simulink model "Filter_data"  (R2025b)
settings: Solver=VariableStepAuto  StartTime=0.0  StopTime=1000  RelTol=1e-3
settings Model: Creator=user  LastModifiedBy=user

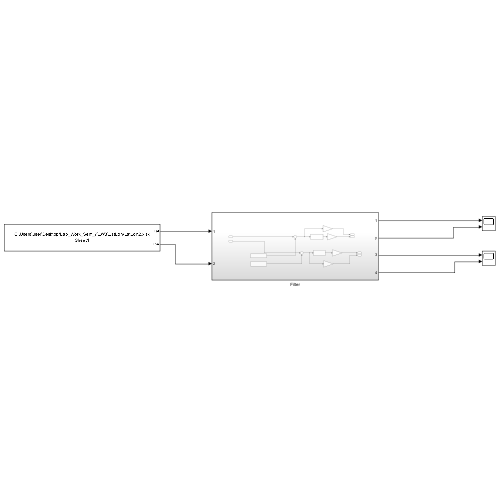
[thumbnail: Simulink's stored preview of the top-level diagram]
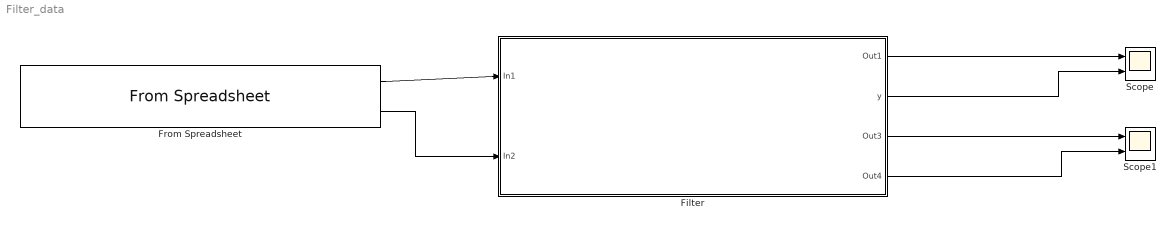
== system Filter_data ==
  Filter : Subsystem
  From Spreadsheet : FromSpreadsheet  FileName=C:\Users\user\Desktop\Lab_Work_Sem_7\LW3\LatLon\LatLon2.xlsx
  Scope : Scope  NumInputPorts=2
      settings: ActiveDisplayYMinimum=-0.22676819893149508  ActiveDisplayYMaximum=2.0409137903834562
  Scope1 : Scope  NumInputPorts=2
      settings: ActiveDisplayYMinimum=-9.25020012785229  ActiveDisplayYMaximum=4.2371666948008748
  wires:
  From Spreadsheet/1 -> Filter/1(In1)
  From Spreadsheet/2 -> Filter/2(In2)
  Filter/1(Out1) -> Scope/1
  Filter/2(y) -> Scope/2
  Filter/3(Out3) -> Scope1/1
  Filter/4(Out4) -> Scope1/2

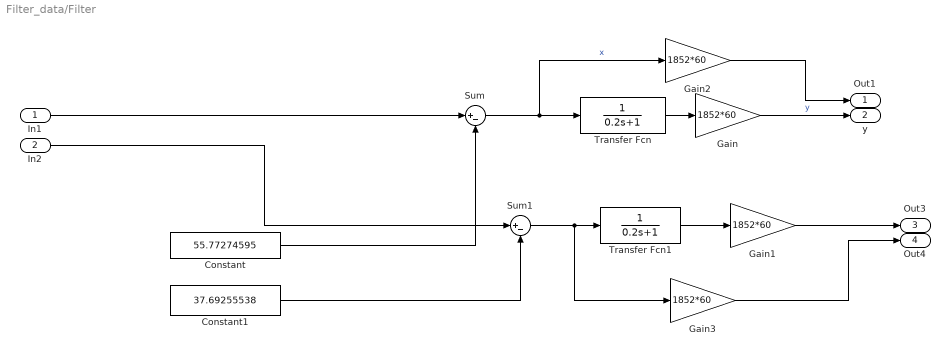
== system Filter_data/Filter ==
  In1 : Inport
  In2 : Inport  Port=2
  Constant : Constant  Value=55.77274595
  Constant1 : Constant  Value=37.69255538
  Gain{,1..3} (4 alike) : Gain  Gain=1852*60
  Sum : Sum  Inputs=|+-
  Sum1 : Sum  Inputs=|+-
  Transfer Fcn : TransferFcn  Denominator=[0.2 1]
  Transfer Fcn1 : TransferFcn  Denominator=[0.2 1]
  Out1 : Outport
  y : Outport  Port=2
  Out3 : Outport  Port=3
  Out4 : Outport  Port=4
  wires:
  Sum1/1 -> Gain3/1, Transfer Fcn1/1
  Transfer Fcn/1 -> Gain/1
  Constant1/1 -> Sum1/2
  Constant/1 -> Sum/2
  Transfer Fcn1/1 -> Gain1/1
  Sum/1 -> Gain2/1, Transfer Fcn/1  "x"
  Gain2/1 -> Out1/1
  In2/1 -> Sum1/1
  Gain1/1 -> Out3/1
  In1/1 -> Sum/1
  Gain/1 -> y/1  "y"
  Gain3/1 -> Out4/1
